simulink model "P3_Variable"  (R2022a)
settings: Solver=VariableStepAuto  StartTime=0.0  StopTime=20  RelTol=1e-3
settings Model: Creator=juanr  LastModifiedBy=juanr

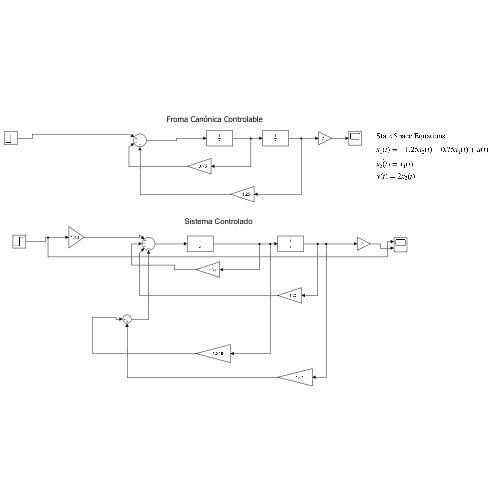
[thumbnail: Simulink's stored preview of the top-level diagram]
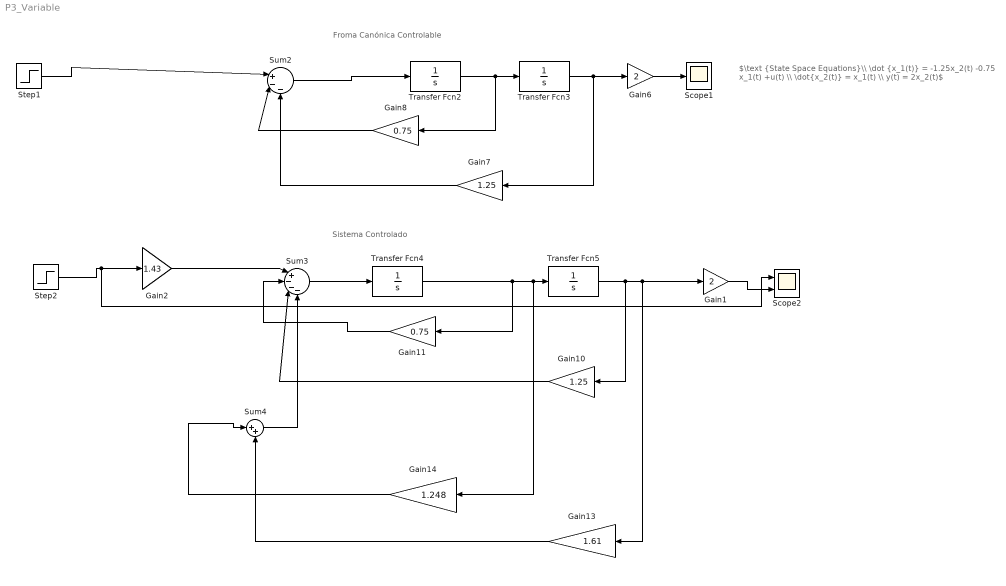
== system P3_Variable ==
  note: Froma Canónica Controlable
  note: $\text {State Space Equations}\\ \dot {x_1(t)} = -1.25x_2(t) -0.75 x_1(t) +u(t) \\ \dot{x_2(t)} = x_1(t) \\ y(t) = 2x_2(t)$
  note: Sistema Controlado
  Gain1 : Gain  Gain=2
  Gain10 : Gain  Gain=1.25
  Gain11 : Gain  Gain=0.75
  Gain13 : Gain  Gain=1.61
  Gain14 : Gain  Gain=1.248
  Gain2 : Gain  Gain=1.43
  Gain6 : Gain  Gain=2
  Gain7 : Gain  Gain=1.25
  Gain8 : Gain  Gain=0.75
  Scope1 : Scope
  Scope2 : Scope  NumInputPorts=2
  Step1 : Step  Time=0  SampleTime=0
  Step2 : Step  Time=0  SampleTime=0.01
  Sum2 : Sum  Inputs=|+--
  Sum3 : Sum  Inputs=|+---
  Sum4 : Sum  Inputs=|++
  Transfer Fcn{2..5} (4 alike) : TransferFcn  Denominator=[1 0]
  wires:
  Transfer Fcn2/1 -> Gain8/1, Transfer Fcn3/1
  Step1/1 -> Sum2/1
  Gain8/1 -> Sum2/2
  Gain7/1 -> Sum2/3
  Transfer Fcn3/1 -> Gain6/1, Gain7/1
  Sum2/1 -> Transfer Fcn2/1
  Sum3/1 -> Transfer Fcn4/1
  Gain10/1 -> Sum3/3
  Sum4/1 -> Sum3/4
  Transfer Fcn4/1 -> Gain14/1, Transfer Fcn5/1, Gain11/1
  Gain11/1 -> Sum3/2
  Gain13/1 -> Sum4/2
  Transfer Fcn5/1 -> Gain1/1, Gain13/1, Gain10/1
  Gain14/1 -> Sum4/1
  Step2/1 -> Scope2/1, Gain2/1
  Gain6/1 -> Scope1/1
  Gain2/1 -> Sum3/1
  Gain1/1 -> Scope2/2
